simulink subsystem "MotionProcessingUnit"  (R2024b)
settings: Solver=VariableStepAuto  StartTime=0.0  StopTime=10.0  RelTol=1e-3
settings Model: Creator=federico  LastModifiedBy=federico

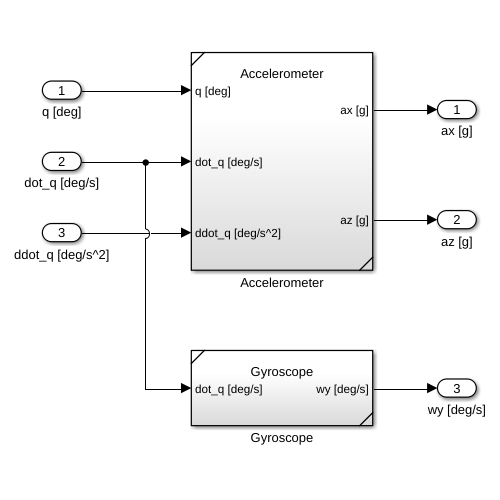
[thumbnail: Simulink's stored preview of the top-level diagram]
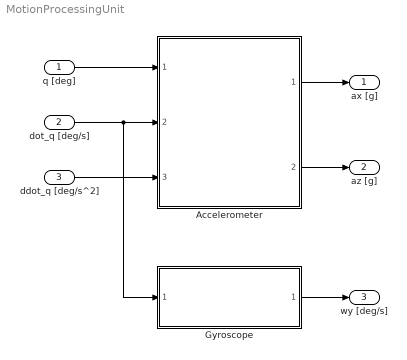
== system MotionProcessingUnit ==
  q [deg] : Inport
  dot_q [deg/s] : Inport  Port=2
  ddot_q [deg/s^2] : Inport  Port=3
  Accelerometer : Subsystem  ReferencedSubsystem=Accelerometer
  Gyroscope : Subsystem  ReferencedSubsystem=Gyroscope
  ax [g] : Outport
  az [g] : Outport  Port=2
  wy [deg/s] : Outport  Port=3
  wires:
  dot_q [deg/s]/1 -> Accelerometer/2, Gyroscope/1
  q [deg]/1 -> Accelerometer/1
  ddot_q [deg/s^2]/1 -> Accelerometer/3
  Accelerometer/1 -> ax [g]/1
  Accelerometer/2 -> az [g]/1
  Gyroscope/1 -> wy [deg/s]/1
